simulink model "packetCat"  (R2015a)
settings: Solver=ode3  StartTime=0.0  StopTime=Inf  FixedStep=0.1  RelTol=1e-3
undefined symbols (not defined in the file): BusSerialize, gcbh, mxpcrtudprx, RigInfo
libraries: xpcnetworkbufferlib x7, xpciplib x5, slrtlib x4, libBusSerialize x2, xpcrtudplib x1
settings Model: xpc_rtwmakecfg_data=_xpcetherlib__xpcether8255xlib__xpcetherGbElib__xpciplib__xpcnblib_  SimulationMode=external  Creator=djoshea  LastModifiedBy=shenoylab
settings SolverCC: EnableConcurrentExecution=on
settings OptimizationCC: BlockReduction=off  OptimizeBlockIOStorage=off  BufferReuse=off  GlobalBufferReuse=off  ExpressionFolding=off  LocalBlockOutputs=off
settings HardwareCC: ProdIntDivRoundTo=Zero  ProdEndianess=LittleEndian  ProdLongLongMode=on  ProdHWDeviceType=Generic->32-bit x86 compatible
settings RTWCC: SystemTargetFile=slrt.tlc  TemplateMakefile=slrt_default_tmf  Description=Simulink Real-Time  RTWCompilerOptimization=on
settings SimulinkRealTimeCC: GeneratePreprocessorConditionals=Disable all

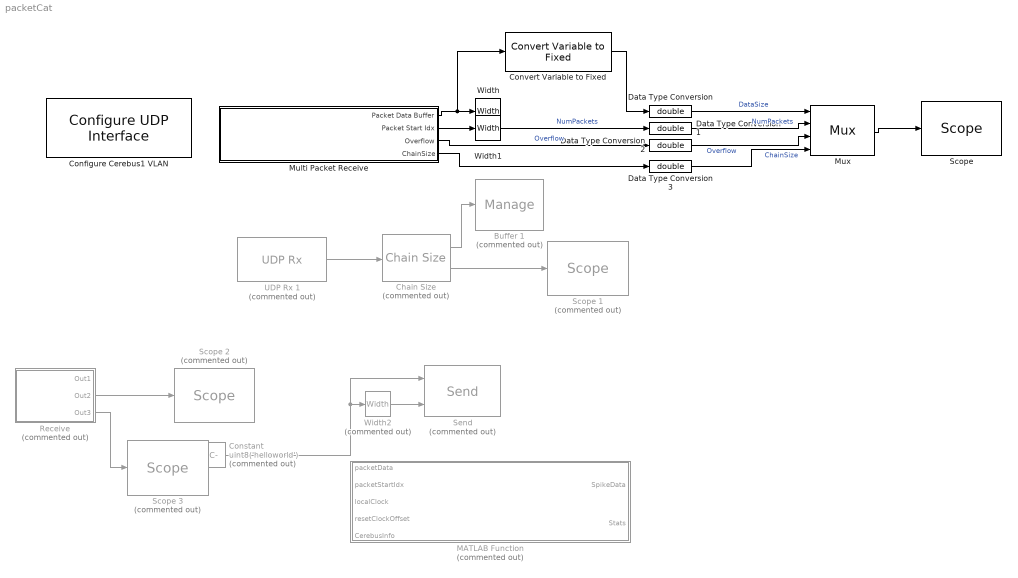
== system packetCat ==
  Buffer 1 : xpcnetworkbufferlib/Manage   Commented=on  ChainSize=0  BufferSize=0  Threshold=0
  "Chain Size " : xpcnetworkbufferlib/Chain Size   Commented=on
  Configure Cerebus1 VLAN : libBusSerialize/Configure UDP Interface  ID=RigInfo.network.cerebus1VLAN.ethernetId  IpAddress=RigInfo.network.cerebus1VLAN.sourceIP  SubnetMask=255.255.255.0  Gateway=0.0.0.0  EthDrv=Intel 8255x  PciBus=RigInfo.network.cerebus1VLAN.pciBus  PciSlot=RigInfo.network.cerebus1VLAN.pciSlot  udpID=0
  Constant : Constant  Commented=on  Value=uint8('helloworld')
  Convert Variable to Fixed : libBusSerialize/Convert Variable to Fixed  bufferSize=1
  Data Type Conversion{,1..3} (4 alike) : DataTypeConversion  OutDataTypeStr=double
  MATLAB Function : MATLAB Function  Commented=on  TreatAsAtomicUnit=on
  "Multi Packet Receive " : Subsystem  InitFcn=mxpcrtudprx(1, get_param(gcbh, 'ID'));  mask(rtudpreceive){ID=RigInfo.network.cerebus1VLAN.ethernetId, sourceIP='0.0.0.0', recvPort=RigInfo.network.cerebus1VLAN.receiveAtPort, PacketDataBufferMaxSize=15000, PacketChainSize=100, PacketBufferSize=0, Receive4=0.1, udpID=0}
      mask prompts: ID "Device ID:"; sourceIP "Source IP Address:"; recvPort "Local (destination) port:"; PacketDataBufferMaxSize "Packet Data Buffer Max Size:"; PacketChainSize "Packet Chain Size"; PacketBufferSize "Packet Buffer Size"; Receive4 "Sample time:"; udpID "Internal UDP ID:"
      mask help:
      | Receive data over UDP network on a dedicated network interface.
      |
      | This block receives data on the specified local (destination) port. To receive all data sent to this port, set 'Source IP Address' to 0.0.0.0. To receive data sent to this port from a specific remote source, enter the IP address of that source.
      mask init:
      | udpID = ID -1;
      mask Help: eval('xpcdoc(''RT_UDP_RECEIVE'')');
      mask Display:
      | try
      |     disp(sprintf('Multi-UDP Receive\nDevice Id: %d\n%s to port %d', ...
      |         ID, BusSerialize.ipStringFromAddress(sourceIP), recvPort));
      | catch
      |     disp('Multi-UDP Receive');
      | end
      | port_label('output', 1, 'Data');
      | port_label('output', 2, 'Start Idx');
      | port_label('output', 3, 'Overflow');
  Mux : Mux
      settings: DisplayOption=signals
  "Receive " : Subsystem  Commented=on  InitFcn=mxpcrtudprx(1, get_param(gcbh, 'ID'));  mask(rtudpreceive){ID=3, Receive1=0.0.0.0, Receive2=1002, Receive3=1500, Receive4=0.1, udpID=0}
      mask prompts: ID "Device ID:"; Receive1 "Source IP Address:"; Receive2 "Local (destination) port:"; Receive3 "Output port width:"; Receive4 "Sample time:"; udpID "Internal UDP ID:"
      mask help:
      | Receive data over UDP network on a dedicated network interface.
      |
      | This block receives data on the specified local (destination) port. To receive all data sent to this port, set 'Source IP Address' to 0.0.0.0. To receive data sent to this port from a specific remote source, enter the IP address of that source.
      mask init:
      | Receive1 = ipaddr(Receive1);
      | udpID = ID -1;
      | [MaskDisplay] = mxpcrtudprx(2, ID);
      | set_param(gcb, 'MaskDisplay', MaskDisplay);
      mask Help: eval('xpcdoc(''RT_UDP_RECEIVE'')');
      mask TypeOptions ID: 1 | 2 | 3 | 4 | 5 | 6 | 7 | 8
      mask Display:
      | disp('UDP\nReceive\nId: 3');
      | port_label('output', 1, 'Data');
      | port_label('output', 2, 'N');
  "Scope " : slrtlib/Displays and Logging/Scope   scopeno=1  scopetype=Target  autostart=on  viewmode=Graphical sliding  formatstr='%15.6f'  grid=on  ylimits=[0,0]  nosamples=250  noprepostsamples=0  interleave=1  triggermode=FreeRun  triggersignal=1  trigsignalfromport=off  triggerlevel=0.0  triggerslope=Either  triggerscope=1  triggersample=0  filename=data.dat  mode=Lazy  writesize=512  autorestart=off  dynamicfilemode=off  maxwritefilesize=512*1024^2
  Scope 1 : slrtlib/Displays and Logging/Scope   Commented=on  scopeno=1  scopetype=Target  autostart=on  viewmode=Graphical redraw  formatstr='%15.6f'  grid=on  ylimits=[0,0]  nosamples=250  noprepostsamples=0  interleave=1  triggermode=FreeRun  triggersignal=1  trigsignalfromport=off  triggerlevel=0.0  triggerslope=Either  triggerscope=1  triggersample=0  filename=data.dat  mode=Lazy  writesize=512  autorestart=off  dynamicfilemode=off  maxwritefilesize=512*1024^2
  Scope 2 : slrtlib/Displays and Logging/Scope   Commented=on  scopeno=1  scopetype=Target  autostart=on  viewmode=Graphical sliding  formatstr='%15.6f'  grid=on  ylimits=[0,0]  nosamples=250  noprepostsamples=0  interleave=1  triggermode=FreeRun  triggersignal=1  trigsignalfromport=off  triggerlevel=0.0  triggerslope=Either  triggerscope=1  triggersample=0  filename=data.dat  mode=Lazy  writesize=512  autorestart=off  dynamicfilemode=off  maxwritefilesize=512*1024^2
  Scope 3 : slrtlib/Displays and Logging/Scope   Commented=on  scopeno=2  scopetype=Target  autostart=on  viewmode=Graphical sliding  formatstr='%15.6f'  grid=on  ylimits=[0,0]  nosamples=250  noprepostsamples=0  interleave=1  triggermode=FreeRun  triggersignal=1  trigsignalfromport=off  triggerlevel=0.0  triggerslope=Either  triggerscope=1  triggersample=0  filename=data.dat  mode=Lazy  writesize=512  autorestart=off  dynamicfilemode=off  maxwritefilesize=512*1024^2
  "Send " : xpcrtudplib/Send   Commented=on  ID=3  Send1=192.168.137.255  Send2=25000  Send3=24000  Send4=0.001  udpID=0
  UDP Rx 1 : xpciplib/UDP Rx   Priority=5  Commented=on  Group=2  sip=Any  SourceAddress=0.0.0.0  lup=Specify  LocalPort=1001  SampleTime=0.001
  Width : Width
  Width1 : Width
  Width2 : Width  Commented=on
  wires:
  "Multi Packet Receive "/1(Packet Data Buffer) -> Convert Variable to Fixed/1, Width/1
  "Multi Packet Receive "/2(Packet Start Idx) -> Width1/1
  Width1/1 -> Data Type Conversion1/1  "NumPackets"
  "Multi Packet Receive "/3(Overflow) -> Data Type Conversion2/1  "Overflow"
  Mux/1 -> "Scope "/1
  Data Type Conversion/1 -> Mux/1  "DataSize"
  Data Type Conversion1/1 -> Mux/2  "NumPackets"
  Data Type Conversion2/1 -> Mux/3  "Overflow"
  "Multi Packet Receive "/4(ChainSize) -> Data Type Conversion3/1
  Data Type Conversion3/1 -> Mux/4  "ChainSize"
  UDP Rx 1/1 -> "Chain Size "/1
  "Chain Size "/2 -> Scope 1/1
  "Chain Size "/1 -> Buffer 1/1
  Constant/1 -> "Send "/1, Width2/1
  Width2/1 -> "Send "/2
  "Receive "/2(Out2) -> Scope 2/1
  "Receive "/3(Out3) -> Scope 3/1
  Convert Variable to Fixed/1 -> Data Type Conversion/1

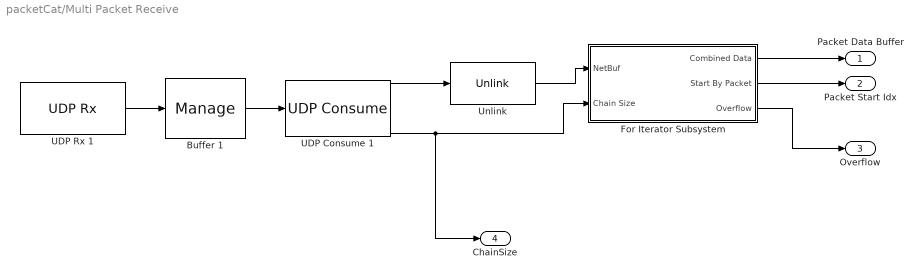
== system packetCat/Multi Packet Receive  ==
  Buffer 1 : xpcnetworkbufferlib/Manage   ChainSize=PacketChainSize  BufferSize=PacketBufferSize  Threshold=0
  For Iterator Subsystem : Subsystem  TreatAsAtomicUnit=on
  UDP Consume 1 : xpciplib/UDP Consume   Group=udpID  VectorSize=PacketChainSize  SampleTime=Receive4
  UDP Rx 1 : xpciplib/UDP Rx   Priority=5  Group=udpID  sip=Any  SourceAddress=BusSerialize.ipAddressFromString(sourceIP)  lup=Specify  LocalPort=recvPort  SampleTime=Receive4
  "Unlink " : xpcnetworkbufferlib/Unlink   VectorLength=PacketChainSize
  Packet Data Buffer : Outport
      settings: VarSizeSig=Yes
  Packet Start Idx : Outport  Port=2
      settings: VarSizeSig=Yes
  Overflow : Outport  Port=3
  ChainSize : Outport  Port=4
  wires:
  UDP Consume 1/6 -> For Iterator Subsystem/2(Chain Size), ChainSize/1
  UDP Consume 1/1 -> "Unlink "/1
  UDP Rx 1/1 -> Buffer 1/1
  Buffer 1/1 -> UDP Consume 1/1
  "Unlink "/1 -> For Iterator Subsystem/1(NetBuf)
  For Iterator Subsystem/1(Combined Data) -> Packet Data Buffer/1
  For Iterator Subsystem/2(Start By Packet) -> Packet Start Idx/1
  For Iterator Subsystem/3(Overflow) -> Overflow/1

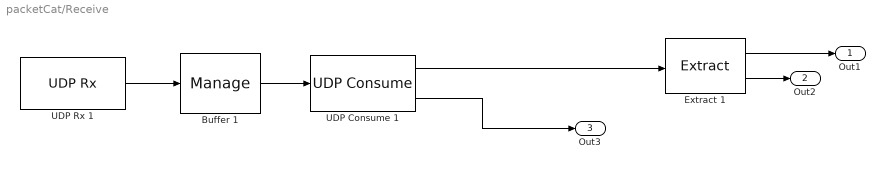
== system packetCat/Receive  ==
  Buffer 1 : xpcnetworkbufferlib/Manage   ChainSize=200  BufferSize=0  Threshold=0
  Extract 1 : xpcnetworkbufferlib/Extract   PacketSize=Receive3
  UDP Consume 1 : xpciplib/UDP Consume   Group=udpID  VectorSize=0  SampleTime=Receive4
  UDP Rx 1 : xpciplib/UDP Rx   Priority=5  Group=2  sip=Any  SourceAddress=0.0.0.0  lup=Specify  LocalPort=1002  SampleTime=0.1
  Out1 : Outport  OutDataTypeStr=uint8
  Out2 : Outport  Port=2  OutDataTypeStr=double
  Out3 : Outport  Port=3
  wires:
  UDP Consume 1/2 -> Out3/1
  UDP Rx 1/1 -> Buffer 1/1
  Buffer 1/1 -> UDP Consume 1/1
  Extract 1/1 -> Out1/1
  Extract 1/2 -> Out2/1
  UDP Consume 1/1 -> Extract 1/1

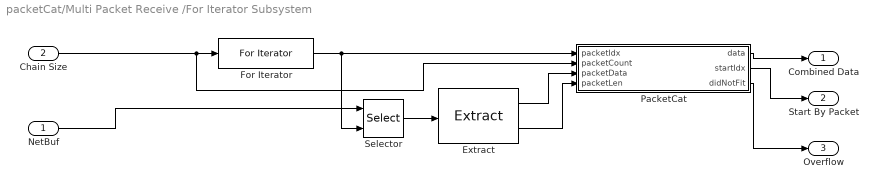
== system packetCat/Multi Packet Receive /For Iterator Subsystem ==
  NetBuf : Inport
  Chain Size : Inport  Port=2
  "Extract " : xpcnetworkbufferlib/Extract   PacketSize=-1
  For Iterator : ForIterator  ResetStates=reset  IterationSource=external
  PacketCat : MATLAB Function  TreatAsAtomicUnit=on
  Selector : Selector  InputPortWidth=PacketChainSize  IndexOptions=Starting index (port)  Indices=[1 3]
  Combined Data : Outport
      settings: VarSizeSig=Yes
  Start By Packet : Outport  Port=2
      settings: VarSizeSig=Yes
  Overflow : Outport  Port=3  OutDataTypeStr=uint8
  wires:
  NetBuf/1 -> Selector/1
  Chain Size/1 -> PacketCat/2(packetCount), For Iterator/1
  For Iterator/1 -> Selector/2, PacketCat/1(packetIdx)
  Selector/1 -> "Extract "/1
  "Extract "/1 -> PacketCat/3(packetData)
  "Extract "/2 -> PacketCat/4(packetLen)
  PacketCat/1(data) -> Combined Data/1
  PacketCat/2(startIdx) -> Start By Packet/1
  PacketCat/3(didNotFit) -> Overflow/1

== matlab function packetCat/MATLAB Function ==
  data: packetData input; SpikeData output; packetStartIdx input; localClock input; resetClockOffset input; CerebusInfo input; Stats output
function [SpikeData, Stats] = parseCerebusPackets(packetData, packetStartIdx, localClock, resetClockOffset, CerebusInfo)

== matlab function packetCat/Multi Packet Receive /For Iterator Subsystem/PacketCat ==
  data: packetIdx input; packetCount input; data output uint8 size=PacketDataBufferMaxSize; packetData input uint8; packetLen input size=1; startIdx output size=PacketChainSize; PacketDataBufferMaxSize parameter size=1; PacketChainSize parameter size=1; didNotFit output uint8 size=1
function [data, startIdx, didNotFit] = packetCat(packetIdx, packetCount, packetData, packetLen, PacketDataBufferMaxSize, PacketChainSize)
%#codegen

persistent pData;
persistent pDataLen;
persistent pStartIdx;
persistent pStartIdxLen;
persistent pDidNotFit;

if packetIdx == 1 || isempty(pData) || isempty(pDataLen) || isempty(pStartIdx) || isempty(pStartIdxLen) || isempty(pDidNotFit)
    pData = coder.nullcopy(zeros(PacketDataBufferMaxSize, 1, 'uint8'));
    pDataLen = uint32(0);
    pStartIdx = coder.nullcopy(zeros(PacketChainSize, 1, 'uint32'));
    pStartIdxLen = uint16(0);
    pDidNotFit = uint8(0);
end

% check whether there is room for this packet
canFitBytes = numel(pData) - pDataLen >= packetLen;
canFitPacket = numel(pStartIdx) - pStartIdxLen > 0;
if canFitBytes && canFitPacket
    % log the start position of this packet
    packetNum = pStartIdxLen + uint16(1);
    pStartIdx(packetNum) = pDataLen + uint32(1);
    pStartIdxLen = pStartIdxLen + 1;
    
    assert(packetLen <= PacketDataBufferMaxSize);
    
    % and copy this packet into the buffer
    dataIdx = pDataLen + uint32(1:packetLen);
    pData(dataIdx) = packetData(uint32(1:packetLen));
    pDataLen = pDataLen + packetLen;
else
    pDidNotFit = uint8(1);
end

if packetIdx == packetCount
    data = pData(1:pDataLen);
    startIdx = pStartIdx(1:pStartIdxLen);
    didNotFit = pDidNotFit;
else
    data = zeros(0, 1, 'uint8');
    startIdx =  zeros(0, 1, 'uint32');
    didNotFit = uint8(0);
end
   
data = uint8(packetLen);
